simulink model "Observer_Arij"  (R2018b)
settings: Solver=VariableStepAuto  StartTime=0.0  StopTime=10.0  RelTol=1e-3
settings Model: Creator=shahidyaqoob  LastModifiedBy=shahidyaqoob

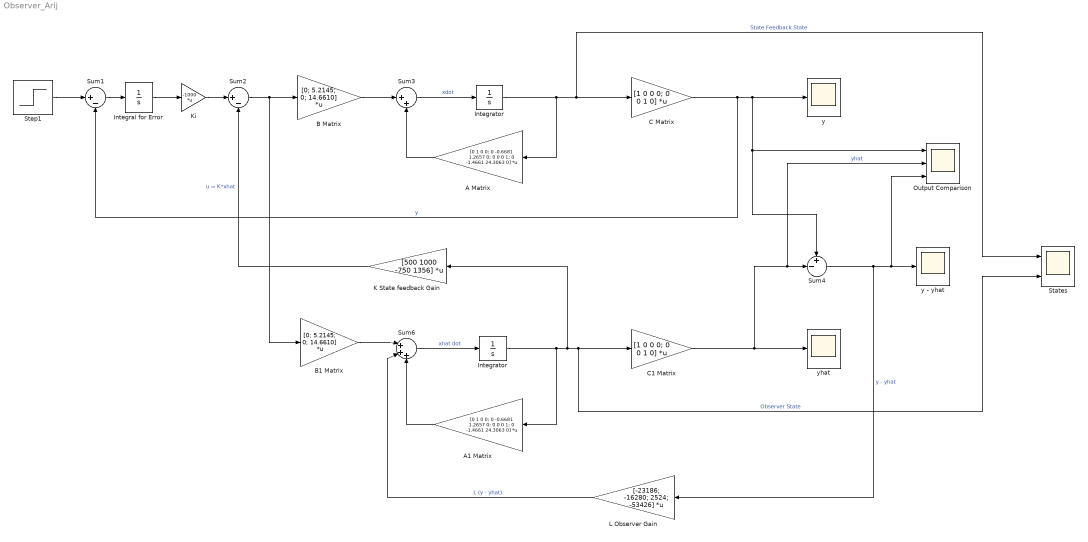
== system Observer_Arij ==
  A Matrix : Gain  Gain=[0 1 0 0; 0 -0.6681 1.2657 0; 0 0 0 1; 0 -1.4661 24.3063 0]  Multiplication=Matrix(K*u)
  A1 Matrix : Gain  Gain=[0 1 0 0; 0 -0.6681 1.2657 0; 0 0 0 1; 0 -1.4661 24.3063 0]  Multiplication=Matrix(K*u)
  B Matrix : Gain  Gain=[0; 5.2145; 0; 14.6610]  Multiplication=Matrix(K*u)
  B1 Matrix : Gain  Gain=[0; 5.2145; 0; 14.6610]  Multiplication=Matrix(K*u)
  C Matrix : Gain  Gain=[1 0 0 0; 0 0 1 0]  Multiplication=Matrix(K*u)
  C1 Matrix : Gain  Gain=[1 0 0 0; 0 0 1 0]  Multiplication=Matrix(K*u)
  Integral for Error : Integrator
  "Integrator " : Integrator  InitialCondition=[0 0 0 ]
  "Integrator " : Integrator  InitialCondition=[0 0 0]
  K State feedback Gain : Gain  Gain=[500 1000 -750 1356]  Multiplication=Matrix(K*u)
  Ki : Gain  Gain=-1000  Multiplication=Matrix(K*u)
  L Observer Gain : Gain  Gain=[-23186; -16280; 2524; -53426]  Multiplication=Matrix(K*u)
  Output Comparison : Scope  NumInputPorts=3
  States : Scope  NumInputPorts=2
  Step1 : Step  Time=0  SampleTime=0
  Sum1 : Sum  Inputs=|+-
  Sum2 : Sum  Inputs=|+-
  Sum3 : Sum  Inputs=|++
  Sum4 : Sum  Inputs=+-|
  Sum6 : Sum  Inputs=|+++
  y : Scope
  y - yhat : Scope
  yhat : Scope
  wires:
  K State feedback Gain/1 -> Sum2/2  "u = K*xhat"
  Sum1/1 -> Integral for Error/1
  Sum6/1 -> "Integrator "/1  "xhat dot"
  Step1/1 -> Sum1/1
  A Matrix/1 -> Sum3/2
  Integral for Error/1 -> Ki/1
  C Matrix/1 -> Output Comparison/1, Sum4/1, y/1, Sum1/2  "y"
  "Integrator "/1 -> C1 Matrix/1, States/2, K State feedback Gain/1, A1 Matrix/1  "Observer State"
  Ki/1 -> Sum2/1
  B Matrix/1 -> Sum3/1
  Sum3/1 -> "Integrator "/1  "xdot"
  "Integrator "/1 -> A Matrix/1, C Matrix/1, States/1  "State Feedback State"
  Sum2/1 -> B Matrix/1, B1 Matrix/1
  B1 Matrix/1 -> Sum6/1
  L Observer Gain/1 -> Sum6/2  "L (y - yhat)"
  C1 Matrix/1 -> yhat/1, Output Comparison/2, Sum4/2  "yhat"
  Sum4/1 -> Output Comparison/3, y - yhat/1, L Observer Gain/1  "y - yhat"
  A1 Matrix/1 -> Sum6/3
